simulink model "testing1"  (R2021a)
settings: Solver=FixedStepDiscrete  StartTime=0.0  StopTime=50  FixedStep=1  RelTol=1e-3
libraries: simulink x2
settings Model: Creator=Rahul  LastModifiedBy=Rahul

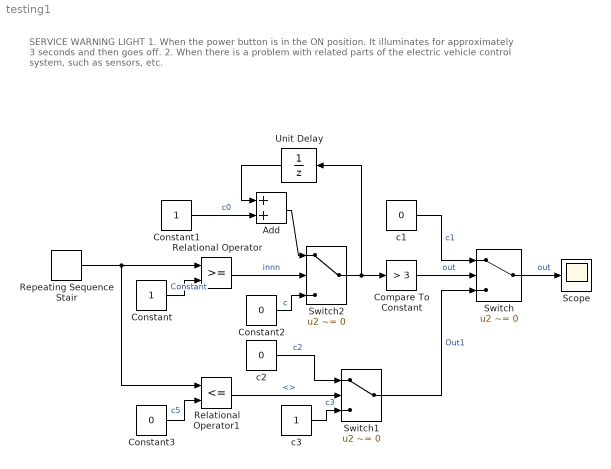
== system testing1 ==
  note: SERVICE WARNING LIGHT
      | 1. When the power button is in the ON position.
      | It illuminates for approximately 3 seconds and then goes off.
      | 2. When there is a problem with related parts of the electric vehicle control system, such as sensors, etc.
  Add : Sum
  Compare To Constant : simulink/Logic and Bit Operations/Compare To Constant  relop=>  const=3  OutDataTypeStr=boolean
  Constant : Constant
  Constant1 : Constant
  Constant2 : Constant  Value=0
  Constant3 : Constant  Value=0
  Relational Operator : RelationalOperator  OutDataTypeStr=boolean  RndMeth=Simplest
  Relational Operator1 : RelationalOperator  Operator=<=  OutDataTypeStr=boolean  RndMeth=Simplest
  Repeating Sequence Stair : simulink/Sources/Repeating Sequence Stair  OutValues=[1 1 1 1 0 0 0 1 1 1 1 0 0 0]  tsamp=-1  OutMin=[]  OutMax=[]  OutDataTypeStr=double  OutputDataTypeScalingMode=double  OutDataType=fixdt(0,8)  ConRadixGroup=Best Precision: Vector-wise  OutScaling=2^-12
  Scope : Scope
  Switch : Switch  Criteria=u2 ~= 0
  Switch1 : Switch  Criteria=u2 ~= 0
  Switch2 : Switch  Criteria=u2 ~= 0
  Unit Delay : UnitDelay  SampleTime=-1  HasFrameUpgradeWarning=on
  c1 : Constant  Value=0
  c2 : Constant  Value=0
  c3 : Constant
  wires:
  Constant1/1 -> Add/2  "c0"
  Relational Operator/1 -> Switch2/2  "innn"
  Unit Delay/1 -> Add/1
  Switch2/1 -> Unit Delay/1, Compare To Constant/1
  Constant2/1 -> Switch2/3  "c"
  Constant/1 -> Relational Operator/2  "Constant"
  Add/1 -> Switch2/1
  Compare To Constant/1 -> Switch/2  "out"
  Constant3/1 -> Relational Operator1/2  "c5"
  Switch1/1 -> Switch/3  "Out1"
  c2/1 -> Switch1/1  "c2"
  Repeating Sequence Stair/1 -> Relational Operator1/1, Relational Operator/1
  c3/1 -> Switch1/3  "c3"
  Relational Operator1/1 -> Switch1/2  "<>"
  Switch/1 -> Scope/1  "out"
  c1/1 -> Switch/1  "c1"
